simulink library "ammclib_bam_S32K3xx"  (R2016a)
settings: Solver=VariableStepAuto  SolverMode=SingleTasking  StartTime=0.0  StopTime=10.0  RelTol=1e-3
undefined symbols (not defined in the file or in its folder): a1, a2, ADCMaxError, autoCalcEn, b0, b1, b2, cfg, dgain, escale, f16A1, f16A2, f16ADCMaxError, f16B0, f16B1, f16B2, f16C1, f16CC1sc, f16CC1sc_D, f16CC1sc_Q, f16CC2sc, f16CC2sc_D, f16CC2sc_Q, f16DerivGain, f16EGain, f16FiltCoef, f16HystOff, f16HystOn, f16IGain, f16IntegGain, f16IntegGain_D, f16IntegGain_Q, f16IntegGainQ, f16Kd, f16KLs, f16Kq, f16KRs, f16Limit, f16LowerLimit, f16LowerLimit_D, f16LowerLimit_Q, f16LowerLimitQ, f16ModIndex, f16OutValOff, f16OutValOn, f16PropGain, f16PropGain_D, f16PropGain_Q, f16PropGainQ, f16RampDown, f16RampUp, f16UGain, f16UpperLimit, f16UpperLimit_D, f16UpperLimit_Q, f16UpperLimitQ, f16WIGain, f32A1, f32A2, f32ADCMaxError ... (+180)
(part 45 of 50)

== system ammclib_bam_S32K3xx/AMCLIB/FLT/AMCLIB_CurrentLoopPIp_FLT ==
  fltUDcBus : Inport  OutDataTypeStr=single  SampleTime=SampleTime
  pIDQReq : Inport  Port=2  OutDataTypeStr=Bus: SWLIBS_2Syst_FLT  SampleTime=SampleTime  BusOutputAsStruct=on
  pIDQFbck : Inport  Port=3  OutDataTypeStr=Bus: SWLIBS_2Syst_FLT  SampleTime=SampleTime  BusOutputAsStruct=on
  fltControllerPIpAWDOut_preset : Inport  Port=4  OutDataTypeStr=single  SampleTime=SampleTime
  fltControllerPIpAWQOut_preset : Inport  Port=5  OutDataTypeStr=single  SampleTime=SampleTime
  Reset : ResetPort  DisableCoverage=on
  AMCLIB_CurrentLoopPIp_SF : S-Function  FunctionName=AMCLIB_CurrentLoopPIp_SF_FLT  Parameters=showStates,resetStatesEnable,fltPropGain_D,fltIntegGain_D,fltPropGain_Q,fltIntegGain_Q,if0,iksi,Ld,Lq,Rs,autoCalcEn  SFunctionDeploymentMode=off  EnableBusSupport=off
  copyright : Subsystem
      mask Display: text(10,90,'FILE:');text(10,75,'DESRIPTION:');text(10,60,'COPYRIGHT:');text(10,45,'VERSION:');text(10,30,'DATE:')
  copyright2 : Subsystem
      mask Display: text(10,90,'AMCLIB_CurrentLoopPIp_BAM_FLT.slx');text(10,75,'PMSM Current Loop.');text(10,60,'NXP 2022');text(10,45,'1.0');text(10,30,'20-Apr-2022');
  fltInK_1_D : Ground
  fltInK_1_D_Out : Terminator
  fltInK_1_Q : Ground
  fltInK_1_Q_Out : Terminator
  fltIntegGain_D : Ground
  fltIntegGain_Q : Ground
  fltIntegPartK_1_D : Ground
  fltIntegPartK_1_D_Out : Terminator
  fltIntegPartK_1_Q : Ground
  fltIntegPartK_1_Q_Out : Terminator
  fltPropGain_D : Ground
  fltPropGain_Q : Ground
  pUDQReq : Outport
  fltUQLim : Outport  Port=2
  wires:
  AMCLIB_CurrentLoopPIp_SF/6 -> fltInK_1_Q_Out/1
  AMCLIB_CurrentLoopPIp_SF/5 -> fltIntegPartK_1_Q_Out/1
  AMCLIB_CurrentLoopPIp_SF/4 -> fltInK_1_D_Out/1
  AMCLIB_CurrentLoopPIp_SF/3 -> fltIntegPartK_1_D_Out/1
  AMCLIB_CurrentLoopPIp_SF/2 -> fltUQLim/1
  AMCLIB_CurrentLoopPIp_SF/1 -> pUDQReq/1
  fltInK_1_Q/1 -> AMCLIB_CurrentLoopPIp_SF/13
  fltIntegPartK_1_Q/1 -> AMCLIB_CurrentLoopPIp_SF/12
  fltIntegGain_Q/1 -> AMCLIB_CurrentLoopPIp_SF/11
  fltPropGain_Q/1 -> AMCLIB_CurrentLoopPIp_SF/10
  fltInK_1_D/1 -> AMCLIB_CurrentLoopPIp_SF/9
  fltIntegPartK_1_D/1 -> AMCLIB_CurrentLoopPIp_SF/8
  fltIntegGain_D/1 -> AMCLIB_CurrentLoopPIp_SF/7
  fltPropGain_D/1 -> AMCLIB_CurrentLoopPIp_SF/6
  fltControllerPIpAWQOut_preset/1 -> AMCLIB_CurrentLoopPIp_SF/5
  fltControllerPIpAWDOut_preset/1 -> AMCLIB_CurrentLoopPIp_SF/4
  pIDQFbck/1 -> AMCLIB_CurrentLoopPIp_SF/3
  pIDQReq/1 -> AMCLIB_CurrentLoopPIp_SF/2
  fltUDcBus/1 -> AMCLIB_CurrentLoopPIp_SF/1

== system ammclib_bam_S32K3xx/AMCLIB/FLT/AMCLIB_CurrentLoop_FLT ==
  fltUDcBus : Inport  OutDataTypeStr=single  SampleTime=SampleTime
  pIDQReq : Inport  Port=2  OutDataTypeStr=Bus: SWLIBS_2Syst_FLT  SampleTime=SampleTime  BusOutputAsStruct=on
  pIDQFbck : Inport  Port=3  OutDataTypeStr=Bus: SWLIBS_2Syst_FLT  SampleTime=SampleTime  BusOutputAsStruct=on
  fltControllerPIrAWDOut_preset : Inport  Port=4  OutDataTypeStr=single  SampleTime=SampleTime
  fltControllerPIrAWQOut_preset : Inport  Port=5  OutDataTypeStr=single  SampleTime=SampleTime
  Reset : ResetPort  DisableCoverage=on
  AMCLIB_CurrentLoop_SF : S-Function  FunctionName=AMCLIB_CurrentLoop_SF_FLT  Parameters=showStates,resetStatesEnable,fltCC1sc_D,fltCC2sc_D,fltCC1sc_Q,fltCC2sc_Q,intmethod,if0,iksi,Ld,Lq,Rs,autoCalcEn  SFunctionDeploymentMode=off  EnableBusSupport=off
  copyright : Subsystem
      mask Display: text(10,90,'FILE:');text(10,75,'DESRIPTION:');text(10,60,'COPYRIGHT:');text(10,45,'VERSION:');text(10,30,'DATE:')
  copyright2 : Subsystem
      mask Display: text(10,90,'AMCLIB_CurrentLoop_BAM_FLT.slx');text(10,75,'PMSM Current Loop.');text(10,60,'NXP 2022');text(10,45,'1.0');text(10,30,'20-Apr-2022');
  fltAcc_D : Ground
  fltAcc_D_Out : Terminator
  fltAcc_Q : Ground
  fltAcc_Q_Out : Terminator
  fltCC1sc_D : Ground
  fltCC1sc_Q : Ground
  fltCC2sc_D : Ground
  fltCC2sc_Q : Ground
  fltInErrK1_D : Ground
  fltInErrK1_D_Out : Terminator
  fltInErrK1_Q : Ground
  fltInErrK1_Q_Out : Terminator
  pUDQReq : Outport
  fltUQLim : Outport  Port=2
  wires:
  AMCLIB_CurrentLoop_SF/6 -> fltInErrK1_Q_Out/1
  AMCLIB_CurrentLoop_SF/5 -> fltAcc_Q_Out/1
  AMCLIB_CurrentLoop_SF/4 -> fltInErrK1_D_Out/1
  AMCLIB_CurrentLoop_SF/3 -> fltAcc_D_Out/1
  AMCLIB_CurrentLoop_SF/2 -> fltUQLim/1
  AMCLIB_CurrentLoop_SF/1 -> pUDQReq/1
  fltInErrK1_Q/1 -> AMCLIB_CurrentLoop_SF/13
  fltAcc_Q/1 -> AMCLIB_CurrentLoop_SF/12
  fltInErrK1_D/1 -> AMCLIB_CurrentLoop_SF/11
  fltAcc_D/1 -> AMCLIB_CurrentLoop_SF/10
  fltCC2sc_Q/1 -> AMCLIB_CurrentLoop_SF/9
  fltCC1sc_Q/1 -> AMCLIB_CurrentLoop_SF/8
  fltCC2sc_D/1 -> AMCLIB_CurrentLoop_SF/7
  fltCC1sc_D/1 -> AMCLIB_CurrentLoop_SF/6
  fltControllerPIrAWQOut_preset/1 -> AMCLIB_CurrentLoop_SF/5
  fltControllerPIrAWDOut_preset/1 -> AMCLIB_CurrentLoop_SF/4
  pIDQFbck/1 -> AMCLIB_CurrentLoop_SF/3
  pIDQReq/1 -> AMCLIB_CurrentLoop_SF/2
  fltUDcBus/1 -> AMCLIB_CurrentLoop_SF/1

== system ammclib_bam_S32K3xx/AMCLIB/FLT/AMCLIB_EstimBJ_FLT ==
  pIAlBeFbck : Inport  OutDataTypeStr=Bus: SWLIBS_2Syst_FLT  BusOutputAsStruct=on
  fltUDcBus : Inport  Port=2  OutDataTypeStr=single
  AMCLIB_EstimBJ_SF : S-Function  FunctionName=AMCLIB_EstimBJ_SF_FLT  Parameters=cfg,u32SamplingFreq,fltIN,fltWN,fltPP,fltLd,fltLq,fltRs,fltDtVDrop,fltAlignTime,fltIReqOl,fltWStepOl,fltDCWReq1,fltDCWReq2,fltDcPiPropGain,fltDcPiIntegGain,fltAcPiPropGain,fltAcPiIntegGain  SFunctionDeploymentMode=off  EnableBusSupport=off
  copyright : Subsystem
      mask Display: text(10,90,'FILE:');text(10,75,'DESRIPTION:');text(10,60,'COPYRIGHT:');text(10,45,'VERSION:');text(10,30,'DATE:')
  copyright2 : Subsystem
      mask Display: text(10,90,'AMCLIB_EstimBJ_BAM_FLT.slx');text(10,75,'PMSM BJ estimator');text(10,60,'NXP 2023');text(10,45,'1.0');text(10,30,'21-Mar-2023');
  returnStatus : Outport
  pUAlBeReq : Outport  Port=2
  fltKt : Outport  Port=3
  fltJ : Outport  Port=4
  fltA : Outport  Port=5
  fltB : Outport  Port=6
  wires:
  AMCLIB_EstimBJ_SF/6 -> fltB/1
  AMCLIB_EstimBJ_SF/5 -> fltA/1
  AMCLIB_EstimBJ_SF/4 -> fltJ/1
  AMCLIB_EstimBJ_SF/3 -> fltKt/1
  AMCLIB_EstimBJ_SF/2 -> pUAlBeReq/1
  AMCLIB_EstimBJ_SF/1 -> returnStatus/1
  fltUDcBus/1 -> AMCLIB_EstimBJ_SF/2
  pIAlBeFbck/1 -> AMCLIB_EstimBJ_SF/1

== system ammclib_bam_S32K3xx/AMCLIB/FLT/AMCLIB_EstimRL_FLT ==
  pIAlBeFbck : Inport  OutDataTypeStr=Bus: SWLIBS_2Syst_FLT  BusOutputAsStruct=on
  fltUDcBus : Inport  Port=2  OutDataTypeStr=single
  fltIDcDReq : Inport  Port=3  OutDataTypeStr=single
  fltIDcQReq : Inport  Port=4  OutDataTypeStr=single
  fltIAcReq : Inport  Port=5  OutDataTypeStr=single
  u16FAc : Inport  Port=6  OutDataTypeStr=uint16
  u8LdqSwitch : Inport  Port=7  OutDataTypeStr=uint8
  AMCLIB_EstimRL_SF : S-Function  FunctionName=AMCLIB_EstimRL_SF_FLT  Parameters=u32SamplingFreq,fltIDcMax,u16LdqNumMeas,fltIDcLd,fltIDcLq,fltIDcNegMax,cfg  SFunctionDeploymentMode=off  EnableBusSupport=off
  copyright : Subsystem
      mask Display: text(10,90,'FILE:');text(10,75,'DESRIPTION:');text(10,60,'COPYRIGHT:');text(10,45,'VERSION:');text(10,30,'DATE:')
  copyright2 : Subsystem
      mask Display: text(10,90,'AMCLIB_EstimRL_BAM_FLT.slx');text(10,75,'PMSM R/Ld/Lq/deadtime estimator');text(10,60,'NXP 2022');text(10,45,'1.0');text(10,30,'20-Apr-2022');
  returnStatus : Outport
  pUAlBeReq : Outport  Port=2
  fltLd : Outport  Port=3
  fltLq : Outport  Port=4
  fltR : Outport  Port=5
  fltUdt : Outport  Port=6
  pLdqTable : Outport  Port=7
  wires:
  AMCLIB_EstimRL_SF/7 -> pLdqTable/1
  AMCLIB_EstimRL_SF/6 -> fltUdt/1
  AMCLIB_EstimRL_SF/5 -> fltR/1
  AMCLIB_EstimRL_SF/4 -> fltLq/1
  AMCLIB_EstimRL_SF/3 -> fltLd/1
  AMCLIB_EstimRL_SF/2 -> pUAlBeReq/1
  AMCLIB_EstimRL_SF/1 -> returnStatus/1
  u8LdqSwitch/1 -> AMCLIB_EstimRL_SF/7
  u16FAc/1 -> AMCLIB_EstimRL_SF/6
  fltIAcReq/1 -> AMCLIB_EstimRL_SF/5
  fltIDcQReq/1 -> AMCLIB_EstimRL_SF/4
  fltIDcDReq/1 -> AMCLIB_EstimRL_SF/3
  fltUDcBus/1 -> AMCLIB_EstimRL_SF/2
  pIAlBeFbck/1 -> AMCLIB_EstimRL_SF/1

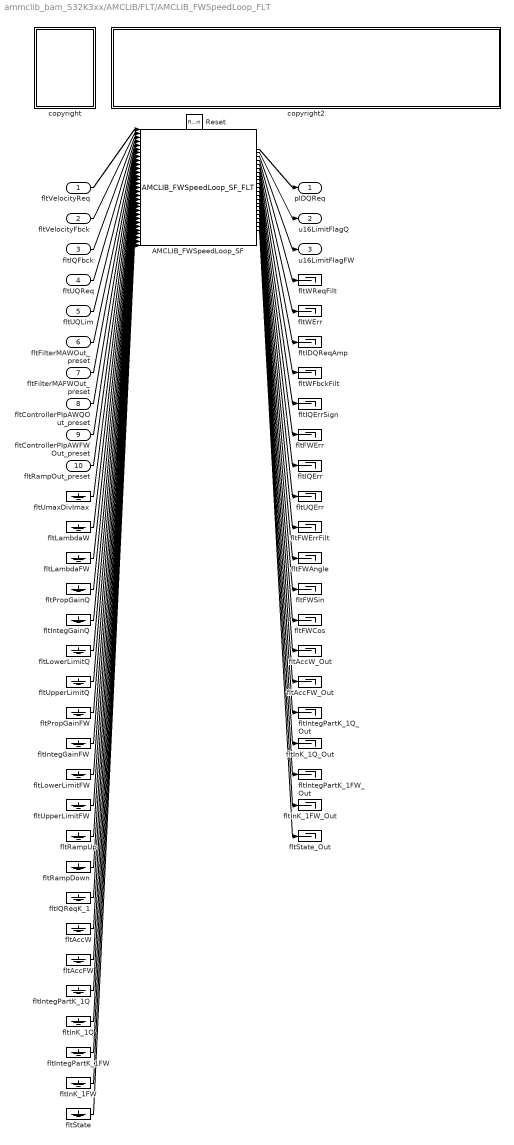
== system ammclib_bam_S32K3xx/AMCLIB/FLT/AMCLIB_FWSpeedLoop_FLT ==
  fltVelocityReq : Inport  OutDataTypeStr=single  SampleTime=SampleTime
  fltVelocityFbck : Inport  Port=2  OutDataTypeStr=single  SampleTime=SampleTime
  fltIQFbck : Inport  Port=3  OutDataTypeStr=single  SampleTime=SampleTime
  fltUQReq : Inport  Port=4  OutDataTypeStr=single  SampleTime=SampleTime
  fltUQLim : Inport  Port=5  OutDataTypeStr=single  SampleTime=SampleTime
  fltFilterMAWOut_preset : Inport  Port=6  OutDataTypeStr=single  SampleTime=SampleTime
  fltFilterMAFWOut_preset : Inport  Port=7  OutDataTypeStr=single  SampleTime=SampleTime
  fltControllerPIpAWQOut_preset : Inport  Port=8  OutDataTypeStr=single  SampleTime=SampleTime
  fltControllerPIpAWFWOut_preset : Inport  Port=9  OutDataTypeStr=single  SampleTime=SampleTime
  fltRampOut_preset : Inport  Port=10  OutDataTypeStr=single  SampleTime=SampleTime
  Reset : ResetPort  DisableCoverage=on
  AMCLIB_FWSpeedLoop_SF : S-Function  FunctionName=AMCLIB_FWSpeedLoop_SF_FLT  Parameters=showStates,resetStatesEnable,showDebugOutputs,fltUmaxDivImax,fltLambdaW,fltLambdaFW,fltPropGainQ,fltIntegGainQ,fltLowerLimitQ,fltUpperLimitQ,fltPropGainFW,fltIntegGainFW,fltLowerLimitFW,fltUpperLimitFW,fltRampUp,fltRampDown,wf0,wksi,J,Kt,lambdaW,lambdaFW,Idmax,imax,udcbus,ramprpm,mechspeed,polepairs,fltState_Out_showOutput,autoCalcEn  SFunctionDeploymentMode=off  EnableBusSupport=off
  copyright : Subsystem
      mask Display: text(10,90,'FILE:');text(10,75,'DESRIPTION:');text(10,60,'COPYRIGHT:');text(10,45,'VERSION:');text(10,30,'DATE:')
  copyright2 : Subsystem
      mask Display: text(10,90,'AMCLIB_FWSpeedLoop_BAM_FLT.slx');text(10,75,'PMSM Speed Loop with Field Weakening.');text(10,60,'NXP 2022');text(10,45,'1.0');text(10,30,'08-Sep-2022');
  fltAccFW : Ground
  fltAccFW_Out : Terminator
  fltAccW : Ground
  fltAccW_Out : Terminator
  fltFWAngle : Terminator
  fltFWCos : Terminator
  fltFWErr : Terminator
  fltFWErrFilt : Terminator
  fltFWSin : Terminator
  fltIDQReqAmp : Terminator
  fltIQErr : Terminator
  fltIQErrSign : Terminator
  fltIQReqK_1 : Ground
  fltInK_1FW : Ground
  fltInK_1FW_Out : Terminator
  fltInK_1Q : Ground
  fltInK_1Q_Out : Terminator
  fltIntegGainFW : Ground
  fltIntegGainQ : Ground
  fltIntegPartK_1FW : Ground
  fltIntegPartK_1FW_Out : Terminator
  fltIntegPartK_1Q : Ground
  fltIntegPartK_1Q_Out : Terminator
  fltLambdaFW : Ground
  fltLambdaW : Ground
  fltLowerLimitFW : Ground
  fltLowerLimitQ : Ground
  fltPropGainFW : Ground
  fltPropGainQ : Ground
  fltRampDown : Ground
  fltRampUp : Ground
  fltState : Ground
  fltState_Out : Terminator
  fltUQErr : Terminator
  fltUmaxDivImax : Ground
  fltUpperLimitFW : Ground
  fltUpperLimitQ : Ground
  fltWErr : Terminator
  fltWFbckFilt : Terminator
  fltWReqFilt : Terminator
  pIDQReq : Outport
  u16LimitFlagQ : Outport  Port=2
  u16LimitFlagFW : Outport  Port=3
  wires:
  AMCLIB_FWSpeedLoop_SF/22 -> fltState_Out/1
  AMCLIB_FWSpeedLoop_SF/21 -> fltInK_1FW_Out/1
  AMCLIB_FWSpeedLoop_SF/20 -> fltIntegPartK_1FW_Out/1
  AMCLIB_FWSpeedLoop_SF/19 -> fltInK_1Q_Out/1
  AMCLIB_FWSpeedLoop_SF/18 -> fltIntegPartK_1Q_Out/1
  AMCLIB_FWSpeedLoop_SF/17 -> fltAccFW_Out/1
  AMCLIB_FWSpeedLoop_SF/16 -> fltAccW_Out/1
  AMCLIB_FWSpeedLoop_SF/15 -> fltFWCos/1
  AMCLIB_FWSpeedLoop_SF/14 -> fltFWSin/1
  AMCLIB_FWSpeedLoop_SF/13 -> fltFWAngle/1
  AMCLIB_FWSpeedLoop_SF/12 -> fltFWErrFilt/1
  AMCLIB_FWSpeedLoop_SF/11 -> fltUQErr/1
  AMCLIB_FWSpeedLoop_SF/10 -> fltIQErr/1
  AMCLIB_FWSpeedLoop_SF/9 -> fltFWErr/1
  AMCLIB_FWSpeedLoop_SF/8 -> fltIQErrSign/1
  AMCLIB_FWSpeedLoop_SF/7 -> fltWFbckFilt/1
  AMCLIB_FWSpeedLoop_SF/6 -> fltIDQReqAmp/1
  AMCLIB_FWSpeedLoop_SF/5 -> fltWErr/1
  AMCLIB_FWSpeedLoop_SF/4 -> fltWReqFilt/1
  AMCLIB_FWSpeedLoop_SF/3 -> u16LimitFlagFW/1
  AMCLIB_FWSpeedLoop_SF/2 -> u16LimitFlagQ/1
  AMCLIB_FWSpeedLoop_SF/1 -> pIDQReq/1
  fltState/1 -> AMCLIB_FWSpeedLoop_SF/31
  fltInK_1FW/1 -> AMCLIB_FWSpeedLoop_SF/30
  fltIntegPartK_1FW/1 -> AMCLIB_FWSpeedLoop_SF/29
  fltInK_1Q/1 -> AMCLIB_FWSpeedLoop_SF/28
  fltIntegPartK_1Q/1 -> AMCLIB_FWSpeedLoop_SF/27
  fltAccFW/1 -> AMCLIB_FWSpeedLoop_SF/26
  fltAccW/1 -> AMCLIB_FWSpeedLoop_SF/25
  fltIQReqK_1/1 -> AMCLIB_FWSpeedLoop_SF/24
  fltRampDown/1 -> AMCLIB_FWSpeedLoop_SF/23
  fltRampUp/1 -> AMCLIB_FWSpeedLoop_SF/22
  fltUpperLimitFW/1 -> AMCLIB_FWSpeedLoop_SF/21
  fltLowerLimitFW/1 -> AMCLIB_FWSpeedLoop_SF/20
  fltIntegGainFW/1 -> AMCLIB_FWSpeedLoop_SF/19
  fltPropGainFW/1 -> AMCLIB_FWSpeedLoop_SF/18
  fltUpperLimitQ/1 -> AMCLIB_FWSpeedLoop_SF/17
  fltLowerLimitQ/1 -> AMCLIB_FWSpeedLoop_SF/16
  fltIntegGainQ/1 -> AMCLIB_FWSpeedLoop_SF/15
  fltPropGainQ/1 -> AMCLIB_FWSpeedLoop_SF/14
  fltLambdaFW/1 -> AMCLIB_FWSpeedLoop_SF/13
  fltLambdaW/1 -> AMCLIB_FWSpeedLoop_SF/12
  fltUmaxDivImax/1 -> AMCLIB_FWSpeedLoop_SF/11
  fltRampOut_preset/1 -> AMCLIB_FWSpeedLoop_SF/10
  fltControllerPIpAWFWOut_preset/1 -> AMCLIB_FWSpeedLoop_SF/9
  fltControllerPIpAWQOut_preset/1 -> AMCLIB_FWSpeedLoop_SF/8
  fltFilterMAFWOut_preset/1 -> AMCLIB_FWSpeedLoop_SF/7
  fltFilterMAWOut_preset/1 -> AMCLIB_FWSpeedLoop_SF/6
  fltUQLim/1 -> AMCLIB_FWSpeedLoop_SF/5
  fltUQReq/1 -> AMCLIB_FWSpeedLoop_SF/4
  fltIQFbck/1 -> AMCLIB_FWSpeedLoop_SF/3
  fltVelocityFbck/1 -> AMCLIB_FWSpeedLoop_SF/2
  fltVelocityReq/1 -> AMCLIB_FWSpeedLoop_SF/1

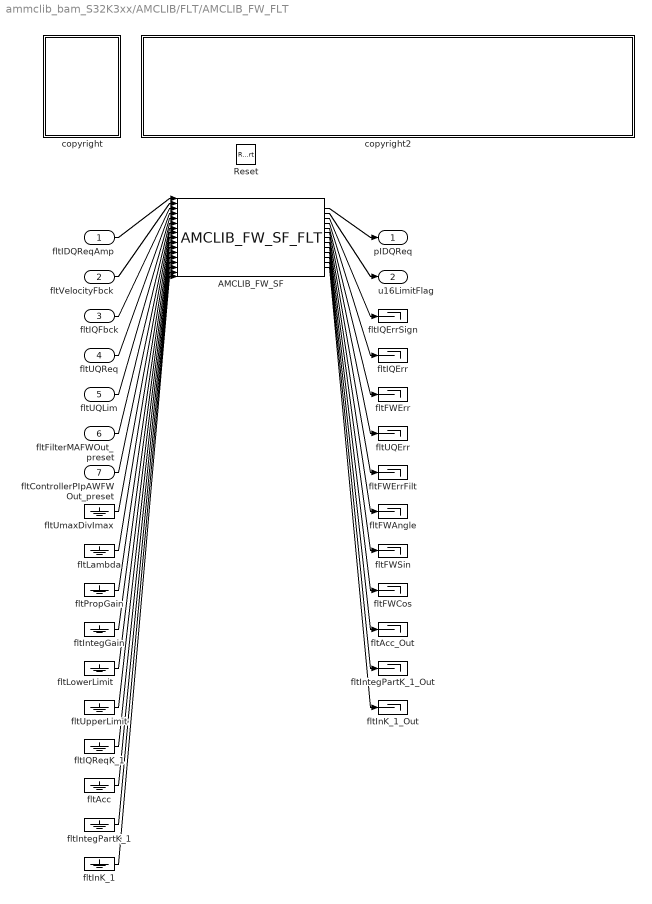
== system ammclib_bam_S32K3xx/AMCLIB/FLT/AMCLIB_FW_FLT ==
  fltIDQReqAmp : Inport  OutDataTypeStr=single  SampleTime=SampleTime
  fltVelocityFbck : Inport  Port=2  OutDataTypeStr=single  SampleTime=SampleTime
  fltIQFbck : Inport  Port=3  OutDataTypeStr=single  SampleTime=SampleTime
  fltUQReq : Inport  Port=4  OutDataTypeStr=single  SampleTime=SampleTime
  fltUQLim : Inport  Port=5  OutDataTypeStr=single  SampleTime=SampleTime
  fltFilterMAFWOut_preset : Inport  Port=6  OutDataTypeStr=single  SampleTime=SampleTime
  fltControllerPIpAWFWOut_preset : Inport  Port=7  OutDataTypeStr=single  SampleTime=SampleTime
  Reset : ResetPort  DisableCoverage=on
  AMCLIB_FW_SF : S-Function  FunctionName=AMCLIB_FW_SF_FLT  Parameters=showStates,resetStatesEnable,showDebugOutputs,fltUmaxDivImax,fltLambda,fltPropGain,fltIntegGain,fltLowerLimit,fltUpperLimit,wf0,wksi,J,Kt,lambdaFW,Idmax,imax,udcbus,autoCalcEn  SFunctionDeploymentMode=off  EnableBusSupport=off
  copyright : Subsystem
      mask Display: text(10,90,'FILE:');text(10,75,'DESRIPTION:');text(10,60,'COPYRIGHT:');text(10,45,'VERSION:');text(10,30,'DATE:')
  copyright2 : Subsystem
      mask Display: text(10,90,'AMCLIB_FW_BAM_FLT.slx');text(10,75,'PMSM Field Weakening Controller');text(10,60,'NXP 2022');text(10,45,'1.0');text(10,30,'20-Apr-2022');
  fltAcc : Ground
  fltAcc_Out : Terminator
  fltFWAngle : Terminator
  fltFWCos : Terminator
  fltFWErr : Terminator
  fltFWErrFilt : Terminator
  fltFWSin : Terminator
  fltIQErr : Terminator
  fltIQErrSign : Terminator
  fltIQReqK_1 : Ground
  fltInK_1 : Ground
  fltInK_1_Out : Terminator
  fltIntegGain : Ground
  fltIntegPartK_1 : Ground
  fltIntegPartK_1_Out : Terminator
  fltLambda : Ground
  fltLowerLimit : Ground
  fltPropGain : Ground
  fltUQErr : Terminator
  fltUmaxDivImax : Ground
  fltUpperLimit : Ground
  pIDQReq : Outport
  u16LimitFlag : Outport  Port=2
  wires:
  AMCLIB_FW_SF/13 -> fltInK_1_Out/1
  AMCLIB_FW_SF/12 -> fltIntegPartK_1_Out/1
  AMCLIB_FW_SF/11 -> fltAcc_Out/1
  AMCLIB_FW_SF/10 -> fltFWCos/1
  AMCLIB_FW_SF/9 -> fltFWSin/1
  AMCLIB_FW_SF/8 -> fltFWAngle/1
  AMCLIB_FW_SF/7 -> fltFWErrFilt/1
  AMCLIB_FW_SF/6 -> fltUQErr/1
  AMCLIB_FW_SF/5 -> fltFWErr/1
  AMCLIB_FW_SF/4 -> fltIQErr/1
  AMCLIB_FW_SF/3 -> fltIQErrSign/1
  AMCLIB_FW_SF/2 -> u16LimitFlag/1
  AMCLIB_FW_SF/1 -> pIDQReq/1
  fltInK_1/1 -> AMCLIB_FW_SF/17
  fltIntegPartK_1/1 -> AMCLIB_FW_SF/16
  fltAcc/1 -> AMCLIB_FW_SF/15
  fltIQReqK_1/1 -> AMCLIB_FW_SF/14
  fltUpperLimit/1 -> AMCLIB_FW_SF/13
  fltLowerLimit/1 -> AMCLIB_FW_SF/12
  fltIntegGain/1 -> AMCLIB_FW_SF/11
  fltPropGain/1 -> AMCLIB_FW_SF/10
  fltLambda/1 -> AMCLIB_FW_SF/9
  fltUmaxDivImax/1 -> AMCLIB_FW_SF/8
  fltControllerPIpAWFWOut_preset/1 -> AMCLIB_FW_SF/7
  fltFilterMAFWOut_preset/1 -> AMCLIB_FW_SF/6
  fltUQLim/1 -> AMCLIB_FW_SF/5
  fltUQReq/1 -> AMCLIB_FW_SF/4
  fltIQFbck/1 -> AMCLIB_FW_SF/3
  fltVelocityFbck/1 -> AMCLIB_FW_SF/2
  fltIDQReqAmp/1 -> AMCLIB_FW_SF/1

== system ammclib_bam_S32K3xx/AMCLIB/FLT/AMCLIB_FluxEstimAB_FLT ==
  fltVelocity : Inport  OutDataTypeStr=single
  pIAB : Inport  Port=2  OutDataTypeStr=Bus: SWLIBS_2Syst_FLT  BusOutputAsStruct=on
  pUAB : Inport  Port=3  OutDataTypeStr=Bus: SWLIBS_2Syst_FLT  BusOutputAsStruct=on
  AMCLIB_FluxEstimAB_SF : S-Function  FunctionName=AMCLIB_FluxEstimAB_SF_FLT  Parameters=showStates,fltRs,fltLs  SFunctionDeploymentMode=off  EnableBusSupport=off
  copyright : Subsystem
      mask Display: text(10,90,'FILE:');text(10,75,'DESRIPTION:');text(10,60,'COPYRIGHT:');text(10,45,'VERSION:');text(10,30,'DATE:')
  copyright2 : Subsystem
      mask Display: text(10,90,'AMCLIB_FluxEstimAB_BAM_FLT.slx');text(10,75,'Rotor flux estimation in Alpha-Beta reference frame.');text(10,60,'NXP 2022');text(10,45,'1.0');text(10,30,'20-Apr-2022');
  fltLs : Ground
  fltRs : Ground
  fltPhase : Outport
  wires:
  AMCLIB_FluxEstimAB_SF/1 -> fltPhase/1
  fltLs/1 -> AMCLIB_FluxEstimAB_SF/5
  fltRs/1 -> AMCLIB_FluxEstimAB_SF/4
  pUAB/1 -> AMCLIB_FluxEstimAB_SF/3
  pIAB/1 -> AMCLIB_FluxEstimAB_SF/2
  fltVelocity/1 -> AMCLIB_FluxEstimAB_SF/1

== system ammclib_bam_S32K3xx/AMCLIB/FLT/AMCLIB_SpeedLoop_FLT ==
  fltVelocityReq : Inport  OutDataTypeStr=single  SampleTime=SampleTime
  fltVelocityFbck : Inport  Port=2  OutDataTypeStr=single  SampleTime=SampleTime
  fltFilterMAWOut_preset : Inport  Port=3  OutDataTypeStr=single  SampleTime=SampleTime
  fltControllerPIpAWQOut_preset : Inport  Port=4  OutDataTypeStr=single  SampleTime=SampleTime
  fltRampOut_preset : Inport  Port=5  OutDataTypeStr=single  SampleTime=SampleTime
  Reset : ResetPort  DisableCoverage=on
  AMCLIB_SpeedLoop_SF : S-Function  FunctionName=AMCLIB_SpeedLoop_SF_FLT  Parameters=showStates,resetStatesEnable,showDebugOutputs,fltLambdaW,fltPropGainQ,fltIntegGainQ,fltLowerLimitQ,fltUpperLimitQ,fltRampUp,fltRampDown,wf0,wksi,J,Kt,lambdaW,ramprpm,mechspeed,polepairs,fltState_Out_showOutput,autoCalcEn  SFunctionDeploymentMode=off  EnableBusSupport=off
  copyright : Subsystem
      mask Display: text(10,90,'FILE:');text(10,75,'DESRIPTION:');text(10,60,'COPYRIGHT:');text(10,45,'VERSION:');text(10,30,'DATE:')
  copyright2 : Subsystem
      mask Display: text(10,90,'AMCLIB_SpeedLoop_BAM_FLT.slx');text(10,75,'PMSM Speed Loop Controller.');text(10,60,'NXP 2022');text(10,45,'1.0');text(10,30,'08-Sep-2022');
  fltAccW : Ground
  fltAccW_Out : Terminator
  fltInK_1Q : Ground
  fltInK_1Q_Out : Terminator
  fltIntegGainQ : Ground
  fltIntegPartK_1Q : Ground
  fltIntegPartK_1Q_Out : Terminator
  fltLambdaW : Ground
  fltLowerLimitQ : Ground
  fltPropGainQ : Ground
  fltRampDown : Ground
  fltRampUp : Ground
  fltState : Ground
  fltState_Out : Terminator
  fltUpperLimitQ : Ground
  fltWErr : Terminator
  fltWFbckFilt : Terminator
  fltWReqFilt : Terminator
  pIDQReq : Outport
  u16LimitFlagQ : Outport  Port=2
  wires:
  AMCLIB_SpeedLoop_SF/9 -> fltState_Out/1
  AMCLIB_SpeedLoop_SF/8 -> fltInK_1Q_Out/1
  AMCLIB_SpeedLoop_SF/7 -> fltIntegPartK_1Q_Out/1
  AMCLIB_SpeedLoop_SF/6 -> fltAccW_Out/1
  AMCLIB_SpeedLoop_SF/5 -> fltWFbckFilt/1
  AMCLIB_SpeedLoop_SF/4 -> fltWErr/1
  AMCLIB_SpeedLoop_SF/3 -> fltWReqFilt/1
  AMCLIB_SpeedLoop_SF/2 -> u16LimitFlagQ/1
  AMCLIB_SpeedLoop_SF/1 -> pIDQReq/1
  fltState/1 -> AMCLIB_SpeedLoop_SF/16
  fltInK_1Q/1 -> AMCLIB_SpeedLoop_SF/15
  fltIntegPartK_1Q/1 -> AMCLIB_SpeedLoop_SF/14
  fltAccW/1 -> AMCLIB_SpeedLoop_SF/13
  fltRampDown/1 -> AMCLIB_SpeedLoop_SF/12
  fltRampUp/1 -> AMCLIB_SpeedLoop_SF/11
  fltUpperLimitQ/1 -> AMCLIB_SpeedLoop_SF/10
  fltLowerLimitQ/1 -> AMCLIB_SpeedLoop_SF/9
  fltIntegGainQ/1 -> AMCLIB_SpeedLoop_SF/8
  fltPropGainQ/1 -> AMCLIB_SpeedLoop_SF/7
  fltLambdaW/1 -> AMCLIB_SpeedLoop_SF/6
  fltRampOut_preset/1 -> AMCLIB_SpeedLoop_SF/5
  fltControllerPIpAWQOut_preset/1 -> AMCLIB_SpeedLoop_SF/4
  fltFilterMAWOut_preset/1 -> AMCLIB_SpeedLoop_SF/3
  fltVelocityFbck/1 -> AMCLIB_SpeedLoop_SF/2
  fltVelocityReq/1 -> AMCLIB_SpeedLoop_SF/1

== system ammclib_bam_S32K3xx/AMCLIB/FLT/AMCLIB_TrackObsrv_FLT ==
  fltPhaseErr : Inport  OutDataTypeStr=single  SampleTime=SampleTime
  fltVelocityOut_preset : Inport  Port=2  OutDataTypeStr=single  SampleTime=SampleTime
  fltPosOut_preset : Inport  Port=3  OutDataTypeStr=single  SampleTime=SampleTime
  Reset : ResetPort  DisableCoverage=on
  AMCLIB_TrackObsrv_SF : S-Function  FunctionName=AMCLIB_TrackObsrv_SF_FLT  Parameters=showStates,resetStatesEnable,fltCC1sc,fltCC2sc,fltUpperLimit,fltLowerLimit,fltC1,intmethod,if0,iksi,autoCalcEn  SFunctionDeploymentMode=off  EnableBusSupport=off
  copyright : Subsystem
      mask Display: text(10,90,'FILE:');text(10,75,'DESRIPTION:');text(10,60,'COPYRIGHT:');text(10,45,'VERSION:');text(10,30,'DATE:')
  copyright2 : Subsystem
      mask Display: text(10,90,'AMCLIB_TrackObsrv_BAM_FLT.slx');text(10,75,'Tracking observer');text(10,60,'NXP 2023');text(10,45,'1.0');text(10,30,'10-Mar-2023');
  fltAcc : Ground
  fltAcc_Out : Terminator
  fltC1 : Ground
  fltCC1 : Ground
  fltCC2 : Ground
  fltInErrK1 : Ground
  fltInErrK1_Out : Terminator
  fltInK1 : Ground
  fltInK1_Out : Terminator
  fltLowerLimit : Ground
  fltState : Ground
  fltState_Out : Terminator
  fltUpperLimit : Ground
  pPosEst : Outport
  pVelocityEst : Outport  Port=2
  wires:
  AMCLIB_TrackObsrv_SF/6 -> fltInK1_Out/1
  AMCLIB_TrackObsrv_SF/5 -> fltState_Out/1
  AMCLIB_TrackObsrv_SF/4 -> fltInErrK1_Out/1
  AMCLIB_TrackObsrv_SF/3 -> fltAcc_Out/1
  AMCLIB_TrackObsrv_SF/2 -> pVelocityEst/1
  AMCLIB_TrackObsrv_SF/1 -> pPosEst/1
  fltInK1/1 -> AMCLIB_TrackObsrv_SF/12
  fltState/1 -> AMCLIB_TrackObsrv_SF/11
  fltInErrK1/1 -> AMCLIB_TrackObsrv_SF/10
  fltAcc/1 -> AMCLIB_TrackObsrv_SF/9
  fltC1/1 -> AMCLIB_TrackObsrv_SF/8
  fltLowerLimit/1 -> AMCLIB_TrackObsrv_SF/7
  fltUpperLimit/1 -> AMCLIB_TrackObsrv_SF/6
  fltCC2/1 -> AMCLIB_TrackObsrv_SF/5
  fltCC1/1 -> AMCLIB_TrackObsrv_SF/4
  fltPosOut_preset/1 -> AMCLIB_TrackObsrv_SF/3
  fltVelocityOut_preset/1 -> AMCLIB_TrackObsrv_SF/2
  fltPhaseErr/1 -> AMCLIB_TrackObsrv_SF/1

== system ammclib_bam_S32K3xx/AMCLIB/FLT/AMCLIB_Windmilling_FLT ==
  pUabcIn : Inport  OutDataTypeStr=Bus: SWLIBS_3Syst_FLT  SampleTime=SampleTime  BusOutputAsStruct=on
  AMCLIB_Windmilling_SF : S-Function  FunctionName=AMCLIB_Windmilling_SF_FLT  Parameters=showStates,fltADCMaxError,fltCC1sc,fltCC2sc,fltUpperLimit,fltLowerLimit,fltC1,if0,iksi,ADCMaxError,autoCalcEn  SFunctionDeploymentMode=off  EnableBusSupport=off
  copyright : Subsystem
      mask Display: text(10,90,'FILE:');text(10,75,'DESRIPTION:');text(10,60,'COPYRIGHT:');text(10,45,'VERSION:');text(10,30,'DATE:')
  copyright2 : Subsystem
      mask Display: text(10,90,'AMCLIB_Windmilling_BAM_FLT.slx');text(10,75,'PMSM Windmilling');text(10,60,'NXP 2022');text(10,45,'1.0');text(10,30,'20-Apr-2022');
  fltADCMaxError : Ground
  fltAccPI : Ground
  fltAccPI_Out : Terminator
  fltC1 : Ground
  fltCC1sc : Ground
  fltCC2sc : Ground
  fltInErrK1 : Ground
  fltInErrK1_Out : Terminator
  fltInK1 : Ground
  fltInK1_Out : Terminator
  fltLowerLimit : Ground
  fltState : Ground
  fltState_Out : Terminator
  fltUpperLimit : Ground
  u32Lock : Outport
  pPosEst : Outport  Port=2
  pVelocityEst : Outport  Port=3
  wires:
  AMCLIB_Windmilling_SF/7 -> fltInK1_Out/1
  AMCLIB_Windmilling_SF/6 -> fltState_Out/1
  AMCLIB_Windmilling_SF/5 -> fltInErrK1_Out/1
  AMCLIB_Windmilling_SF/4 -> fltAccPI_Out/1
  AMCLIB_Windmilling_SF/3 -> pVelocityEst/1
  AMCLIB_Windmilling_SF/2 -> pPosEst/1
  AMCLIB_Windmilling_SF/1 -> u32Lock/1
  fltInK1/1 -> AMCLIB_Windmilling_SF/11
  fltState/1 -> AMCLIB_Windmilling_SF/10
  fltInErrK1/1 -> AMCLIB_Windmilling_SF/9
  fltAccPI/1 -> AMCLIB_Windmilling_SF/8
  fltC1/1 -> AMCLIB_Windmilling_SF/7
  fltLowerLimit/1 -> AMCLIB_Windmilling_SF/6
  fltUpperLimit/1 -> AMCLIB_Windmilling_SF/5
  fltCC2sc/1 -> AMCLIB_Windmilling_SF/4
  fltCC1sc/1 -> AMCLIB_Windmilling_SF/3
  fltADCMaxError/1 -> AMCLIB_Windmilling_SF/2
  pUabcIn/1 -> AMCLIB_Windmilling_SF/1

== system ammclib_bam_S32K3xx/GDFLIB/F16/GDFLIB_FilterFIR_F16 ==
  f16In : Inport  OutDataTypeStr=int16
  GDFLIB_FilterFIR_SF : S-Function  FunctionName=GDFLIB_FilterFIR_SF_F16  Parameters=u16Order,pCoefBuf  SFunctionDeploymentMode=off  EnableBusSupport=off
  copyright : Subsystem
      mask Display: text(10,90,'FILE:');text(10,75,'DESRIPTION:');text(10,60,'COPYRIGHT:');text(10,45,'VERSION:');text(10,30,'DATE:')
  copyright2 : Subsystem
      mask Display: text(10,90,'GDFLIB_FilterFIR_BAM_F16.slx');text(10,75,'FIR filter.');text(10,60,'NXP 2022');text(10,45,'1.0');text(10,30,'20-Apr-2022');
  f16Out : Outport
  wires:
  GDFLIB_FilterFIR_SF/1 -> f16Out/1
  f16In/1 -> GDFLIB_FilterFIR_SF/1

== system ammclib_bam_S32K3xx/GDFLIB/F16/GDFLIB_FilterIIR1_F16 ==
  f16In : Inport  OutDataTypeStr=int16
  GDFLIB_FilterIIR1_SF : S-Function  FunctionName=GDFLIB_FilterIIR1_SF_F16  Parameters=showStates,f16B0,f16B1,f16A1,b0,b1,a1,autoCalcEn  SFunctionDeploymentMode=off  EnableBusSupport=off
  copyright : Subsystem
      mask Display: text(10,90,'FILE:');text(10,75,'DESRIPTION:');text(10,60,'COPYRIGHT:');text(10,45,'VERSION:');text(10,30,'DATE:')
  copyright2 : Subsystem
      mask Display: text(10,90,'GDFLIB_FilterIIR1_BAM_F16.slx');text(10,75,'First order IIR filter.');text(10,60,'NXP 2022');text(10,45,'1.0');text(10,30,'20-Apr-2022');
  f16A1 : Ground
  f16B0 : Ground
  f16B1 : Ground
  f16FiltBufferX : Ground
  f16FiltBufferX_Out : Terminator
  f32FiltBufferY : Ground
  f32FiltBufferY_Out : Terminator
  f16Out : Outport
  wires:
  GDFLIB_FilterIIR1_SF/3 -> f32FiltBufferY_Out/1
  GDFLIB_FilterIIR1_SF/2 -> f16FiltBufferX_Out/1
  GDFLIB_FilterIIR1_SF/1 -> f16Out/1
  f32FiltBufferY/1 -> GDFLIB_FilterIIR1_SF/6
  f16FiltBufferX/1 -> GDFLIB_FilterIIR1_SF/5
  f16A1/1 -> GDFLIB_FilterIIR1_SF/4
  f16B1/1 -> GDFLIB_FilterIIR1_SF/3
  f16B0/1 -> GDFLIB_FilterIIR1_SF/2
  f16In/1 -> GDFLIB_FilterIIR1_SF/1

== system ammclib_bam_S32K3xx/GDFLIB/F16/GDFLIB_FilterIIR2_F16 ==
  f16In : Inport  OutDataTypeStr=int16
  FilterBufferX1_Out : Terminator
  FilterBufferX2_Out : Terminator
  FilterBufferY1_Out : Terminator
  FilterBufferY2_Out : Terminator
  GDFLIB_FilterIIR2_SF : S-Function  FunctionName=GDFLIB_FilterIIR2_SF_F16  Parameters=showStates,f16B0,f16B1,f16B2,f16A1,f16A2,b0,b1,b2,a1,a2,autoCalcEn  SFunctionDeploymentMode=off  EnableBusSupport=off
  copyright : Subsystem
      mask Display: text(10,90,'FILE:');text(10,75,'DESRIPTION:');text(10,60,'COPYRIGHT:');text(10,45,'VERSION:');text(10,30,'DATE:')
  copyright2 : Subsystem
      mask Display: text(10,90,'GDFLIB_FilterIIR2_BAM_F16.slx');text(10,75,'First order IIR filter.');text(10,60,'NXP 2022');text(10,45,'1.0');text(10,30,'20-Apr-2022');
  f16A1 : Ground
  f16A2 : Ground
  f16B0 : Ground
  f16B1 : Ground
  f16B2 : Ground
  f16FiltBufferX1 : Ground
  f16FiltBufferX2 : Ground
  f32FiltBufferY1 : Ground
  f32FiltBufferY2 : Ground
  f16Out : Outport
  wires:
  GDFLIB_FilterIIR2_SF/5 -> FilterBufferY2_Out/1
  GDFLIB_FilterIIR2_SF/4 -> FilterBufferY1_Out/1
  GDFLIB_FilterIIR2_SF/3 -> FilterBufferX2_Out/1
  GDFLIB_FilterIIR2_SF/2 -> FilterBufferX1_Out/1
  GDFLIB_FilterIIR2_SF/1 -> f16Out/1
  f16A2/1 -> GDFLIB_FilterIIR2_SF/10
  f16A1/1 -> GDFLIB_FilterIIR2_SF/9
  f16B2/1 -> GDFLIB_FilterIIR2_SF/8
  f16B1/1 -> GDFLIB_FilterIIR2_SF/7
  f16B0/1 -> GDFLIB_FilterIIR2_SF/6
  f32FiltBufferY2/1 -> GDFLIB_FilterIIR2_SF/5
  f32FiltBufferY1/1 -> GDFLIB_FilterIIR2_SF/4
  f16FiltBufferX2/1 -> GDFLIB_FilterIIR2_SF/3
  f16FiltBufferX1/1 -> GDFLIB_FilterIIR2_SF/2
  f16In/1 -> GDFLIB_FilterIIR2_SF/1

== system ammclib_bam_S32K3xx/GDFLIB/F16/GDFLIB_FilterMA_F16 ==
  f16In : Inport  OutDataTypeStr=int16
  f16FilterMAOut_preset : Inport  Port=2  OutDataTypeStr=int16
  Reset : ResetPort  DisableCoverage=on
  GDFLIB_FilterMA_SF : S-Function  FunctionName=GDFLIB_FilterMA_SF_F16  Parameters=showStates,resetStatesEnable,u16NSamples  SFunctionDeploymentMode=off  EnableBusSupport=off
  copyright : Subsystem
      mask Display: text(10,90,'FILE:');text(10,75,'DESRIPTION:');text(10,60,'COPYRIGHT:');text(10,45,'VERSION:');text(10,30,'DATE:')
  copyright2 : Subsystem
      mask Display: text(10,90,'GDFLIB_FilterMA_BAM_F16.slx');text(10,75,'Exponential moving average filter.');text(10,60,'NXP 2022');text(10,45,'1.0');text(10,30,'20-Apr-2022');
  f32Acc : Ground
  f32Acc_Out : Terminator
  u16NSamples : Ground
  f16Out : Outport
  wires:
  GDFLIB_FilterMA_SF/2 -> f32Acc_Out/1
  GDFLIB_FilterMA_SF/1 -> f16Out/1
  f32Acc/1 -> GDFLIB_FilterMA_SF/4
  u16NSamples/1 -> GDFLIB_FilterMA_SF/3
  f16FilterMAOut_preset/1 -> GDFLIB_FilterMA_SF/2
  f16In/1 -> GDFLIB_FilterMA_SF/1

== system ammclib_bam_S32K3xx/GDFLIB/F32/GDFLIB_FilterFIR_F32 ==
  f32In : Inport  OutDataTypeStr=int32
  GDFLIB_FilterFIR_SF : S-Function  FunctionName=GDFLIB_FilterFIR_SF_F32  Parameters=u32Order,pCoefBuf  SFunctionDeploymentMode=off  EnableBusSupport=off
  copyright : Subsystem
      mask Display: text(10,90,'FILE:');text(10,75,'DESRIPTION:');text(10,60,'COPYRIGHT:');text(10,45,'VERSION:');text(10,30,'DATE:')
  copyright2 : Subsystem
      mask Display: text(10,90,'GDFLIB_FilterFIR_BAM_F32.slx');text(10,75,'FIR filter.');text(10,60,'NXP 2022');text(10,45,'1.0');text(10,30,'20-Apr-2022');
  f32Out : Outport
  wires:
  GDFLIB_FilterFIR_SF/1 -> f32Out/1
  f32In/1 -> GDFLIB_FilterFIR_SF/1

== system ammclib_bam_S32K3xx/GDFLIB/F32/GDFLIB_FilterIIR1_F32 ==
  f32In : Inport  OutDataTypeStr=int32
  GDFLIB_FilterIIR1_SF : S-Function  FunctionName=GDFLIB_FilterIIR1_SF_F32  Parameters=showStates,f32B0,f32B1,f32A1,b0,b1,a1,autoCalcEn  SFunctionDeploymentMode=off  EnableBusSupport=off
  copyright : Subsystem
      mask Display: text(10,90,'FILE:');text(10,75,'DESRIPTION:');text(10,60,'COPYRIGHT:');text(10,45,'VERSION:');text(10,30,'DATE:')
  copyright2 : Subsystem
      mask Display: text(10,90,'GDFLIB_FilterIIR1_BAM_F32.slx');text(10,75,'First order IIR filter.');text(10,60,'NXP 2022');text(10,45,'1.0');text(10,30,'20-Apr-2022');
  f32A1 : Ground
  f32B0 : Ground
  f32B1 : Ground
  f32FiltBufferX : Ground
  f32FiltBufferX_Out : Terminator
  f32FiltBufferY : Ground
  f32FiltBufferY_Out : Terminator
  f32Out : Outport
  wires:
  GDFLIB_FilterIIR1_SF/3 -> f32FiltBufferY_Out/1
  GDFLIB_FilterIIR1_SF/2 -> f32FiltBufferX_Out/1
  GDFLIB_FilterIIR1_SF/1 -> f32Out/1
  f32FiltBufferY/1 -> GDFLIB_FilterIIR1_SF/6
  f32FiltBufferX/1 -> GDFLIB_FilterIIR1_SF/5
  f32A1/1 -> GDFLIB_FilterIIR1_SF/4
  f32B1/1 -> GDFLIB_FilterIIR1_SF/3
  f32B0/1 -> GDFLIB_FilterIIR1_SF/2
  f32In/1 -> GDFLIB_FilterIIR1_SF/1

== system ammclib_bam_S32K3xx/GDFLIB/F32/GDFLIB_FilterIIR2_F32 ==
  f32In : Inport  OutDataTypeStr=int32
  FilterBufferX1_Out : Terminator
  FilterBufferX2_Out : Terminator
  FilterBufferY1_Out : Terminator
  FilterBufferY2_Out : Terminator
  GDFLIB_FilterIIR2_SF : S-Function  FunctionName=GDFLIB_FilterIIR2_SF_F32  Parameters=showStates,f32B0,f32B1,f32B2,f32A1,f32A2,b0,b1,b2,a1,a2,autoCalcEn  SFunctionDeploymentMode=off  EnableBusSupport=off
  copyright : Subsystem
      mask Display: text(10,90,'FILE:');text(10,75,'DESRIPTION:');text(10,60,'COPYRIGHT:');text(10,45,'VERSION:');text(10,30,'DATE:')
  copyright2 : Subsystem
      mask Display: text(10,90,'GDFLIB_FilterIIR2_BAM_F32.slx');text(10,75,'First order IIR filter.');text(10,60,'NXP 2022');text(10,45,'1.0');text(10,30,'20-Apr-2022');
  f32A1 : Ground
  f32A2 : Ground
  f32B0 : Ground
  f32B1 : Ground
  f32B2 : Ground
  f32FiltBufferX1 : Ground
  f32FiltBufferX2 : Ground
  f32FiltBufferY1 : Ground
  f32FiltBufferY2 : Ground
  f32Out : Outport
  wires:
  GDFLIB_FilterIIR2_SF/5 -> FilterBufferY2_Out/1
  GDFLIB_FilterIIR2_SF/4 -> FilterBufferY1_Out/1
  GDFLIB_FilterIIR2_SF/3 -> FilterBufferX2_Out/1
  GDFLIB_FilterIIR2_SF/2 -> FilterBufferX1_Out/1
  GDFLIB_FilterIIR2_SF/1 -> f32Out/1
  f32A2/1 -> GDFLIB_FilterIIR2_SF/10
  f32A1/1 -> GDFLIB_FilterIIR2_SF/9
  f32B2/1 -> GDFLIB_FilterIIR2_SF/8
  f32B1/1 -> GDFLIB_FilterIIR2_SF/7
  f32B0/1 -> GDFLIB_FilterIIR2_SF/6
  f32FiltBufferY2/1 -> GDFLIB_FilterIIR2_SF/5
  f32FiltBufferY1/1 -> GDFLIB_FilterIIR2_SF/4
  f32FiltBufferX2/1 -> GDFLIB_FilterIIR2_SF/3
  f32FiltBufferX1/1 -> GDFLIB_FilterIIR2_SF/2
  f32In/1 -> GDFLIB_FilterIIR2_SF/1

== system ammclib_bam_S32K3xx/GDFLIB/F32/GDFLIB_FilterMA_F32 ==
  f32In : Inport  OutDataTypeStr=int32
  f32FilterMAOut_preset : Inport  Port=2  OutDataTypeStr=int32
  Reset : ResetPort  DisableCoverage=on
  GDFLIB_FilterMA_SF : S-Function  FunctionName=GDFLIB_FilterMA_SF_F32  Parameters=showStates,resetStatesEnable,u16NSamples  SFunctionDeploymentMode=off  EnableBusSupport=off
  copyright : Subsystem
      mask Display: text(10,90,'FILE:');text(10,75,'DESRIPTION:');text(10,60,'COPYRIGHT:');text(10,45,'VERSION:');text(10,30,'DATE:')
  copyright2 : Subsystem
      mask Display: text(10,90,'GDFLIB_FilterMA_BAM_F32.slx');text(10,75,'Exponential moving average filter.');text(10,60,'NXP 2022');text(10,45,'1.0');text(10,30,'20-Apr-2022');
  f32Acc : Ground
  f32Acc_Out : Terminator
  u16NSamples : Ground
  f32Out : Outport
  wires:
  GDFLIB_FilterMA_SF/2 -> f32Acc_Out/1
  GDFLIB_FilterMA_SF/1 -> f32Out/1
  f32Acc/1 -> GDFLIB_FilterMA_SF/4
  u16NSamples/1 -> GDFLIB_FilterMA_SF/3
  f32FilterMAOut_preset/1 -> GDFLIB_FilterMA_SF/2
  f32In/1 -> GDFLIB_FilterMA_SF/1

== system ammclib_bam_S32K3xx/GDFLIB/FLT/GDFLIB_FilterFIR_FLT ==
  fltIn : Inport  OutDataTypeStr=single
  GDFLIB_FilterFIR_SF : S-Function  FunctionName=GDFLIB_FilterFIR_SF_FLT  Parameters=u32Order,pCoefBuf  SFunctionDeploymentMode=off  EnableBusSupport=off
  copyright : Subsystem
      mask Display: text(10,90,'FILE:');text(10,75,'DESRIPTION:');text(10,60,'COPYRIGHT:');text(10,45,'VERSION:');text(10,30,'DATE:')
  copyright2 : Subsystem
      mask Display: text(10,90,'GDFLIB_FilterFIR_BAM_FLT.slx');text(10,75,'FIR filter.');text(10,60,'NXP 2022');text(10,45,'1.0');text(10,30,'20-Apr-2022');
  fltOut : Outport
  wires:
  GDFLIB_FilterFIR_SF/1 -> fltOut/1
  fltIn/1 -> GDFLIB_FilterFIR_SF/1

== system ammclib_bam_S32K3xx/GDFLIB/FLT/GDFLIB_FilterIIR1_FLT ==
  fltIn : Inport  OutDataTypeStr=single
  GDFLIB_FilterIIR1_SF : S-Function  FunctionName=GDFLIB_FilterIIR1_SF_FLT  Parameters=showStates,fltB0,fltB1,fltA1  SFunctionDeploymentMode=off  EnableBusSupport=off
  copyright : Subsystem
      mask Display: text(10,90,'FILE:');text(10,75,'DESRIPTION:');text(10,60,'COPYRIGHT:');text(10,45,'VERSION:');text(10,30,'DATE:')
  copyright2 : Subsystem
      mask Display: text(10,90,'GDFLIB_FilterIIR1_BAM_FLT.slx');text(10,75,'First order IIR filter.');text(10,60,'NXP 2022');text(10,45,'1.0');text(10,30,'20-Apr-2022');
  fltA1 : Ground
  fltB0 : Ground
  fltB1 : Ground
  fltFiltBufferX : Ground
  fltFiltBufferX_Out : Terminator
  fltFiltBufferY : Ground
  fltFiltBufferY_Out : Terminator
  fltOut : Outport
  wires:
  GDFLIB_FilterIIR1_SF/3 -> fltFiltBufferY_Out/1
  GDFLIB_FilterIIR1_SF/2 -> fltFiltBufferX_Out/1
  GDFLIB_FilterIIR1_SF/1 -> fltOut/1
  fltFiltBufferY/1 -> GDFLIB_FilterIIR1_SF/6
  fltFiltBufferX/1 -> GDFLIB_FilterIIR1_SF/5
  fltA1/1 -> GDFLIB_FilterIIR1_SF/4
  fltB1/1 -> GDFLIB_FilterIIR1_SF/3
  fltB0/1 -> GDFLIB_FilterIIR1_SF/2
  fltIn/1 -> GDFLIB_FilterIIR1_SF/1

== system ammclib_bam_S32K3xx/GDFLIB/FLT/GDFLIB_FilterIIR2_FLT ==
  fltIn : Inport  OutDataTypeStr=single
  FilterBufferX1_Out : Terminator
  FilterBufferX2_Out : Terminator
  FilterBufferY1_Out : Terminator
  FilterBufferY2_Out : Terminator
  GDFLIB_FilterIIR2_SF : S-Function  FunctionName=GDFLIB_FilterIIR2_SF_FLT  Parameters=showStates,fltB0,fltB1,fltB2,fltA1,fltA2  SFunctionDeploymentMode=off  EnableBusSupport=off
  copyright : Subsystem
      mask Display: text(10,90,'FILE:');text(10,75,'DESRIPTION:');text(10,60,'COPYRIGHT:');text(10,45,'VERSION:');text(10,30,'DATE:')
  copyright2 : Subsystem
      mask Display: text(10,90,'GDFLIB_FilterIIR2_BAM_FLT.slx');text(10,75,'First order IIR filter.');text(10,60,'NXP 2022');text(10,45,'1.0');text(10,30,'20-Apr-2022');
  fltA1 : Ground
  fltA2 : Ground
  fltB0 : Ground
  fltB1 : Ground
  fltB2 : Ground
  fltFiltBufferX1 : Ground
  fltFiltBufferX2 : Ground
  fltFiltBufferY1 : Ground
  fltFiltBufferY2 : Ground
  fltOut : Outport
  wires:
  GDFLIB_FilterIIR2_SF/5 -> FilterBufferY2_Out/1
  GDFLIB_FilterIIR2_SF/4 -> FilterBufferY1_Out/1
  GDFLIB_FilterIIR2_SF/3 -> FilterBufferX2_Out/1
  GDFLIB_FilterIIR2_SF/2 -> FilterBufferX1_Out/1
  GDFLIB_FilterIIR2_SF/1 -> fltOut/1
  fltA2/1 -> GDFLIB_FilterIIR2_SF/10
  fltA1/1 -> GDFLIB_FilterIIR2_SF/9
  fltB2/1 -> GDFLIB_FilterIIR2_SF/8
  fltB1/1 -> GDFLIB_FilterIIR2_SF/7
  fltB0/1 -> GDFLIB_FilterIIR2_SF/6
  fltFiltBufferY2/1 -> GDFLIB_FilterIIR2_SF/5
  fltFiltBufferY1/1 -> GDFLIB_FilterIIR2_SF/4
  fltFiltBufferX2/1 -> GDFLIB_FilterIIR2_SF/3
  fltFiltBufferX1/1 -> GDFLIB_FilterIIR2_SF/2
  fltIn/1 -> GDFLIB_FilterIIR2_SF/1

== system ammclib_bam_S32K3xx/GDFLIB/FLT/GDFLIB_FilterMA_FLT ==
  fltIn : Inport  OutDataTypeStr=single
  fltFilterMAOut_preset : Inport  Port=2  OutDataTypeStr=single
  Reset : ResetPort  DisableCoverage=on
  GDFLIB_FilterMA_SF : S-Function  FunctionName=GDFLIB_FilterMA_SF_FLT  Parameters=showStates,resetStatesEnable,fltLambda  SFunctionDeploymentMode=off  EnableBusSupport=off
  copyright : Subsystem
      mask Display: text(10,90,'FILE:');text(10,75,'DESRIPTION:');text(10,60,'COPYRIGHT:');text(10,45,'VERSION:');text(10,30,'DATE:')
  copyright2 : Subsystem
      mask Display: text(10,90,'GDFLIB_FilterMA_BAM_FLT.slx');text(10,75,'Exponential moving average filter.');text(10,60,'NXP 2022');text(10,45,'1.0');text(10,30,'20-Apr-2022');
  fltAcc : Ground
  fltAcc_Out : Terminator
  fltLambda : Ground
  fltOut : Outport
  wires:
  GDFLIB_FilterMA_SF/2 -> fltAcc_Out/1
  GDFLIB_FilterMA_SF/1 -> fltOut/1
  fltAcc/1 -> GDFLIB_FilterMA_SF/4
  fltLambda/1 -> GDFLIB_FilterMA_SF/3
  fltFilterMAOut_preset/1 -> GDFLIB_FilterMA_SF/2
  fltIn/1 -> GDFLIB_FilterMA_SF/1

== system ammclib_bam_S32K3xx/GFLIB/F16/GFLIB_Acos_F16 ==
  f16In : Inport  OutDataTypeStr=int16
  GFLIB_Acos_SF : S-Function  FunctionName=GFLIB_Acos_SF_F16  SFunctionDeploymentMode=off  EnableBusSupport=off
  copyright : Subsystem
      mask Display: text(10,90,'FILE:');text(10,75,'DESRIPTION:');text(10,60,'COPYRIGHT:');text(10,45,'VERSION:');text(10,30,'DATE:')
  copyright2 : Subsystem
      mask Display: text(10,90,'GFLIB_Acos_BAM_F16.slx');text(10,75,'Inverse cosine function');text(10,60,'NXP 2022');text(10,45,'1.0');text(10,30,'20-Apr-2022');
  f16Out : Outport
  wires:
  GFLIB_Acos_SF/1 -> f16Out/1
  f16In/1 -> GFLIB_Acos_SF/1

== system ammclib_bam_S32K3xx/GFLIB/F16/GFLIB_Asin_F16 ==
  f16In : Inport  OutDataTypeStr=int16
  GFLIB_Asin_SF : S-Function  FunctionName=GFLIB_Asin_SF_F16  SFunctionDeploymentMode=off  EnableBusSupport=off
  copyright : Subsystem
      mask Display: text(10,90,'FILE:');text(10,75,'DESRIPTION:');text(10,60,'COPYRIGHT:');text(10,45,'VERSION:');text(10,30,'DATE:')
  copyright2 : Subsystem
      mask Display: text(10,90,'GFLIB_Asin_BAM_F16.slx');text(10,75,'Inverse sine function');text(10,60,'NXP 2022');text(10,45,'1.0');text(10,30,'20-Apr-2022');
  f16Out : Outport
  wires:
  GFLIB_Asin_SF/1 -> f16Out/1
  f16In/1 -> GFLIB_Asin_SF/1

== system ammclib_bam_S32K3xx/GFLIB/F16/GFLIB_AtanYXShifted_F16 ==
  f16InY : Inport  OutDataTypeStr=int16
  f16InX : Inport  Port=2  OutDataTypeStr=int16
  Ky : Inport  Port=3  OutDataTypeStr=int16
  Kx : Inport  Port=4  OutDataTypeStr=int16
  Ny : Inport  Port=5  OutDataTypeStr=int16
  Nx : Inport  Port=6  OutDataTypeStr=int16
  ThetaAdj : Inport  Port=7  OutDataTypeStr=int16
  GFLIB_AtanYXShifted_SF : S-Function  FunctionName=GFLIB_AtanYXShifted_SF_F16  SFunctionDeploymentMode=off  EnableBusSupport=off
  copyright : Subsystem
      mask Display: text(10,90,'FILE:');text(10,75,'DESRIPTION:');text(10,60,'COPYRIGHT:');text(10,45,'VERSION:');text(10,30,'DATE:')
  copyright2 : Subsystem
      mask Display: text(10,90,'GFLIB_AtanYXShifted_BAM_F16.slx');text(10,75,'Shifted arctangent of two arguments Y/X.');text(10,60,'NXP 2022');text(10,45,'1.0');text(10,30,'20-Apr-2022');
  f16Out : Outport
  wires:
  GFLIB_AtanYXShifted_SF/1 -> f16Out/1
  ThetaAdj/1 -> GFLIB_AtanYXShifted_SF/7
  Nx/1 -> GFLIB_AtanYXShifted_SF/6
  Ny/1 -> GFLIB_AtanYXShifted_SF/5
  Kx/1 -> GFLIB_AtanYXShifted_SF/4
  Ky/1 -> GFLIB_AtanYXShifted_SF/3
  f16InX/1 -> GFLIB_AtanYXShifted_SF/2
  f16InY/1 -> GFLIB_AtanYXShifted_SF/1

== system ammclib_bam_S32K3xx/GFLIB/F16/GFLIB_AtanYX_F16 ==
  f16InY : Inport  OutDataTypeStr=int16
  f16InX : Inport  Port=2  OutDataTypeStr=int16
  GFLIB_AtanYX_SF : S-Function  FunctionName=GFLIB_AtanYX_SF_F16  SFunctionDeploymentMode=off  EnableBusSupport=off
  copyright : Subsystem
      mask Display: text(10,90,'FILE:');text(10,75,'DESRIPTION:');text(10,60,'COPYRIGHT:');text(10,45,'VERSION:');text(10,30,'DATE:')
  copyright2 : Subsystem
      mask Display: text(10,90,'GFLIB_AtanYX_BAM_F16.slx');text(10,75,'Arctangent of two arguments Y/X.');text(10,60,'NXP 2022');text(10,45,'1.0');text(10,30,'20-Apr-2022');
  f16Out : Outport
  wires:
  GFLIB_AtanYX_SF/1 -> f16Out/1
  f16InX/1 -> GFLIB_AtanYX_SF/2
  f16InY/1 -> GFLIB_AtanYX_SF/1

== system ammclib_bam_S32K3xx/GFLIB/F16/GFLIB_Atan_F16 ==
  f16In : Inport  OutDataTypeStr=int16
  GFLIB_Atan_SF : S-Function  FunctionName=GFLIB_Atan_SF_F16  SFunctionDeploymentMode=off  EnableBusSupport=off
  copyright : Subsystem
      mask Display: text(10,90,'FILE:');text(10,75,'DESRIPTION:');text(10,60,'COPYRIGHT:');text(10,45,'VERSION:');text(10,30,'DATE:')
  copyright2 : Subsystem
      mask Display: text(10,90,'GFLIB_Atan_BAM_F16.slx');text(10,75,'Inverse tangent function');text(10,60,'NXP 2022');text(10,45,'1.0');text(10,30,'20-Apr-2022');
  f16Out : Outport
  wires:
  GFLIB_Atan_SF/1 -> f16Out/1
  f16In/1 -> GFLIB_Atan_SF/1

== system ammclib_bam_S32K3xx/GFLIB/F16/GFLIB_ControllerPIDpAW_F16 ==
  f16InErr : Inport  OutDataTypeStr=int16  SampleTime=SampleTime
  f16ControllerPIDpAWOut_preset : Inport  Port=2  OutDataTypeStr=int16  SampleTime=SampleTime
  Reset : ResetPort  DisableCoverage=on
  GFLIB_ControllerPIDpAW_SF : S-Function  FunctionName=GFLIB_ControllerPIDpAW_SF_F16  Parameters=showStates,resetStatesEnable,f16PropGain,f16IntegGain,f16DerivGain,f16FiltCoef,s16PropGainShift,s16IntegGainShift,s16DerivGainShift,f16LowerLimit,f16UpperLimit,pgain,igain,dgain,filtCoef,lowerLimit,upperLimit,inscale,outscale,autoCalcEn  SFunctionDeploymentMode=off  EnableBusSupport=off
  copyright : Subsystem
      mask Display: text(10,90,'FILE:');text(10,75,'DESRIPTION:');text(10,60,'COPYRIGHT:');text(10,45,'VERSION:');text(10,30,'DATE:')
  copyright2 : Subsystem
      mask Display: text(10,90,'GFLIB_ControllerPIDpAW_BAM_F16.slx');text(10,75,'Parallel form of a standard PID controller with anti-windup.');text(10,60,'NXP 2022');text(10,45,'1.0');text(10,30,'20-Apr-2022');
  f16DerivGain : Ground
  f16DerivPartK_1 : Ground
  f16DerivPartK_1_Out : Terminator
  f16FiltCoef : Ground
  f16InK_1 : Ground
  f16InK_1_Out : Terminator
  f16IntegGain : Ground
  f16LowerLimit : Ground
  f16PropGain : Ground
  f16UpperLimit : Ground
  f32IntegPartK_1 : Ground
  f32IntegPartK_1_Out : Terminator
  s16DerivGainShift : Ground
  s16IntegGainShift : Ground
  s16PropGainShift : Ground
  f16Out : Outport
  u16LimitFlag : Outport  Port=2
  wires:
  GFLIB_ControllerPIDpAW_SF/5 -> f16InK_1_Out/1
  GFLIB_ControllerPIDpAW_SF/4 -> f16DerivPartK_1_Out/1
  GFLIB_ControllerPIDpAW_SF/3 -> f32IntegPartK_1_Out/1
  GFLIB_ControllerPIDpAW_SF/2 -> u16LimitFlag/1
  GFLIB_ControllerPIDpAW_SF/1 -> f16Out/1
  f16InK_1/1 -> GFLIB_ControllerPIDpAW_SF/14
  f16DerivPartK_1/1 -> GFLIB_ControllerPIDpAW_SF/13
  f32IntegPartK_1/1 -> GFLIB_ControllerPIDpAW_SF/12
  f16UpperLimit/1 -> GFLIB_ControllerPIDpAW_SF/11
  f16LowerLimit/1 -> GFLIB_ControllerPIDpAW_SF/10
  s16DerivGainShift/1 -> GFLIB_ControllerPIDpAW_SF/9
  s16IntegGainShift/1 -> GFLIB_ControllerPIDpAW_SF/8
  s16PropGainShift/1 -> GFLIB_ControllerPIDpAW_SF/7
  f16FiltCoef/1 -> GFLIB_ControllerPIDpAW_SF/6
  f16DerivGain/1 -> GFLIB_ControllerPIDpAW_SF/5
  f16IntegGain/1 -> GFLIB_ControllerPIDpAW_SF/4
  f16PropGain/1 -> GFLIB_ControllerPIDpAW_SF/3
  f16ControllerPIDpAWOut_preset/1 -> GFLIB_ControllerPIDpAW_SF/2
  f16InErr/1 -> GFLIB_ControllerPIDpAW_SF/1

== system ammclib_bam_S32K3xx/GFLIB/F16/GFLIB_ControllerPIpAW_F16 ==
  f16InErr : Inport  OutDataTypeStr=int16  SampleTime=SampleTime
  f16ControllerPIpAWOut_preset : Inport  Port=2  OutDataTypeStr=int16  SampleTime=SampleTime
  Reset : ResetPort  DisableCoverage=on
  GFLIB_ControllerPIpAW_SF : S-Function  FunctionName=GFLIB_ControllerPIpAW_SF_F16  Parameters=showStates,resetStatesEnable,f16PropGain,f16IntegGain,s16PropGainShift,s16IntegGainShift,f16LowerLimit,f16UpperLimit,pgain,igain,lowerLimit,upperLimit,inscale,outscale,autoCalcEn  SFunctionDeploymentMode=off  EnableBusSupport=off
  copyright : Subsystem
      mask Display: text(10,90,'FILE:');text(10,75,'DESRIPTION:');text(10,60,'COPYRIGHT:');text(10,45,'VERSION:');text(10,30,'DATE:')
  copyright2 : Subsystem
      mask Display: text(10,90,'GFLIB_ControllerPIpAW_BAM_F16.slx');text(10,75,'Parallel form of a standard PI controller with anti-windup.');text(10,60,'NXP 2022');text(10,45,'1.0');text(10,30,'20-Apr-2022');
  f16InK_1 : Ground
  f16InK_1_Out : Terminator
  f16IntegGain : Ground
  f16LowerLimit : Ground
  f16PropGain : Ground
  f16UpperLimit : Ground
  f32IntegPartK_1 : Ground
  f32IntegPartK_1_Out : Terminator
  s16IntegGainShift : Ground
  s16PropGainShift : Ground
  f16Out : Outport
  u16LimitFlag : Outport  Port=2
  wires:
  GFLIB_ControllerPIpAW_SF/4 -> f16InK_1_Out/1
  GFLIB_ControllerPIpAW_SF/3 -> f32IntegPartK_1_Out/1
  GFLIB_ControllerPIpAW_SF/2 -> u16LimitFlag/1
  GFLIB_ControllerPIpAW_SF/1 -> f16Out/1
  f16InK_1/1 -> GFLIB_ControllerPIpAW_SF/10
  f32IntegPartK_1/1 -> GFLIB_ControllerPIpAW_SF/9
  f16UpperLimit/1 -> GFLIB_ControllerPIpAW_SF/8
  f16LowerLimit/1 -> GFLIB_ControllerPIpAW_SF/7
  s16IntegGainShift/1 -> GFLIB_ControllerPIpAW_SF/6
  s16PropGainShift/1 -> GFLIB_ControllerPIpAW_SF/5
  f16IntegGain/1 -> GFLIB_ControllerPIpAW_SF/4
  f16PropGain/1 -> GFLIB_ControllerPIpAW_SF/3
  f16ControllerPIpAWOut_preset/1 -> GFLIB_ControllerPIpAW_SF/2
  f16InErr/1 -> GFLIB_ControllerPIpAW_SF/1

== system ammclib_bam_S32K3xx/GFLIB/F16/GFLIB_ControllerPIp_F16 ==
  f16InErr : Inport  OutDataTypeStr=int16  SampleTime=SampleTime
  f16ControllerPIpOut_preset : Inport  Port=2  OutDataTypeStr=int16  SampleTime=SampleTime
  Reset : ResetPort  DisableCoverage=on
  GFLIB_ControllerPIp_SF : S-Function  FunctionName=GFLIB_ControllerPIp_SF_F16  Parameters=showStates,resetStatesEnable,f16PropGain,f16IntegGain,s16PropGainShift,s16IntegGainShift,pgain,igain,inscale,outscale,autoCalcEn  SFunctionDeploymentMode=off  EnableBusSupport=off
  copyright : Subsystem
      mask Display: text(10,90,'FILE:');text(10,75,'DESRIPTION:');text(10,60,'COPYRIGHT:');text(10,45,'VERSION:');text(10,30,'DATE:')
  copyright2 : Subsystem
      mask Display: text(10,90,'GFLIB_ControllerPIp_BAM_F16.slx');text(10,75,'Parallel form of a standard PI controller without anti-windup.');text(10,60,'NXP 2022');text(10,45,'1.0');text(10,30,'20-Apr-2022');
  f16InK_1 : Ground
  f16InK_1_Out : Terminator
  f16IntegGain : Ground
  f16PropGain : Ground
  f32IntegPartK_1 : Ground
  f32IntegPartK_1_Out : Terminator
  s16IntegGainShift : Ground
  s16PropGainShift : Ground
  f16Out : Outport
  wires:
  GFLIB_ControllerPIp_SF/3 -> f16InK_1_Out/1
  GFLIB_ControllerPIp_SF/2 -> f32IntegPartK_1_Out/1
  GFLIB_ControllerPIp_SF/1 -> f16Out/1
  f16InK_1/1 -> GFLIB_ControllerPIp_SF/8
  f32IntegPartK_1/1 -> GFLIB_ControllerPIp_SF/7
  s16IntegGainShift/1 -> GFLIB_ControllerPIp_SF/6
  s16PropGainShift/1 -> GFLIB_ControllerPIp_SF/5
  f16IntegGain/1 -> GFLIB_ControllerPIp_SF/4
  f16PropGain/1 -> GFLIB_ControllerPIp_SF/3
  f16ControllerPIpOut_preset/1 -> GFLIB_ControllerPIp_SF/2
  f16InErr/1 -> GFLIB_ControllerPIp_SF/1
